simulink model "DTMF_Telefonie_Project_Crehul_Hornai"  (R2018b)
settings: Solver=VariableStepAuto  StartTime=0.0  StopTime=100  RelTol=1e-3
undefined symbols (not defined in the file): fdesignblkfcn, gcbh
libraries: simulink x12, dspfdesign x7
(part 2 of 4)

== system DTMF_Telefonie_Project_Crehul_Hornai/DTMF Detector and Decoder/Subsystem/1477Hz Bandpass Filter ==
  In : Inport
  Generated Filter Block : DiscreteFir  Tag=BlockMethodSubSystem  Coefficients=[0.000678764862504704263 0.000804373453114689695 -0.000424094188809401567 0.000167209003489621763 -0.000242270760367763161 4.6470921147658429e-05 6.95206164852695159e-06 0.000136313750795735581 5.73971292841914723e-05 -1.08891135695370588e-05 -0.00010807231843965948 -0.000100678178529028895 -2.39139709179673077e-05 8.22719619307408709e-05 0.000121322031372226961 6.67195498408230687e-05 -4.54322205964575315e-05 -0.000123546441105899405 -0.000105769303813425504 -1.47191102267772017e-06 0.000106642780553394814 0.000132557583534852327 5.13511648645235529e-05 -7.37028057411876717e-05 -0.000143736658268125549 -9.92899356923174822e-05 2.59446525748383179e-05 0.000134079459699696767 0.000136741672296518922 3.01685686462495675e-05 -0.000104187130503145776 -0.000158239484929200433 -8.67404980072451152e-05 5.74174071110912943e-05 0.000158308721508832297 0.000134444966268375916 1.8284919510189266e-06 -0.000134817878355808192 -0.000167440391573942578 -6.55512682525988006e-05 9.14538284917498345e-05 0.000178631042614973241 0.000123874664584542075 -3.05242741126250487e-05 -0.000164714196852270645 -0.000169025187109667335 -3.7701329655403246e-05 0.000126528809334661456 0.000192066158003905601 0.000105799063218011509 -6.79533803345053634e-05 -0.000189773665441093139 -0.000161994152014295189 -3.95880851204494406e-06 0.000160060971546786227 0.000199138171986074433 7.8476057786001311e-05 -0.000105980075455429975 -0.000209346483238170194 -0.000146288941368850336 3.45550752056478314e-05 0.000190352324485544306 0.000196109461443976646 4.54400805598609726e-05 -0.000144484544870355494 -0.000220406187691344485 -0.000121964269468380565 7.58152294997171006e-05 0.00021488709301901044 0.000184083746180164782 5.93982545919963592e-06 -0.000178893689660710982 -0.000223002253409260078 -8.89183572636694994e-05 0.000116458060922216113 0.000231657134855096621 0.000162204277360463367 -3.64712308000864505e-05 -0.000208119503375310717 -0.000214664067654908195 -5.02598167574192737e-05 0.000155096389684706779 0.000238098225791522154 0.000132194115690055384 -7.99892046078015499e-05 -0.000228623801064775992 -0.000196701983237502565 -7.34495975451181574e-06 0.000187575168349489452 0.000234483903146764146 9.4383718966663515e-05 -0.000120350652338928072 -0.00023975742986282909 -0.000168765668975382659 3.62796888475293202e-05 0.000212334960261702623 0.000219332269412665605 5.26832536310174303e-05 -0.000155766501238902705 -0.000239303864982351108 -0.000133517294274330045 7.82814639436078472e-05 0.000226012067649557441 0.000194762278839820174 8.6425324803695875e-06 -0.000182112956171246246 -0.000227689150524581184 -9.25658528431953353e-05 0.000114226987622273067 0.000228657881637320173 0.000161021804288971051 -3.27910592299296682e-05 -0.000198224146624526205 -0.000204801318833720825 -4.99979298250496137e-05 0.000141908848976985986 0.000218455210176687897 0.000122065229315672548 -6.91953924481208526e-05 -0.000201291882550297093 -0.00017324112862875953 -8.77095916717294567e-06 0.000157781157199081944 0.000197131314976748805 8.00474503860715107e-05 -9.56231695524905126e-05 -0.000192124851322154596 -0.000134438958140752031 2.573733020283216e-05 0.000161008172845363701 0.000165063910650344644 4.07422142637717342e-05 -0.000110735349115864516 -0.000169367326537080923 -9.38498835634843289e-05 5.12370725678648956e-05 0.000149182379205609061 0.000126667649759154262 7.12439653057449739e-06 -0.00011079587869896961 -0.000136065294631048609 -5.48549739532533474e-05 6.29644289637935114e-05 0.000123760079219049609 8.49249951684299779e-05 -1.54504623116251492e-05 -9.51766421847845007e-05 -9.47953617583736398e-05 -2.27547304877335002e-05 5.8641671409375264e-05 8.59013188943345395e-05 4.53598683612078338e-05 -2.32918846142151498e-05 -6.37716681334422452e-05 -5.01656451408910315e-05 -2.43092022642965935e-06 3.63407014523718219e-05 3.92725335328120324e-05 1.30810954317975205e-05 -1.28066060299382271e-05 -1.84926479954187692e-05 -7.304766428425577e-06 1.06809246101379103e-06 ...(+19715 chars)]  InputProcessing=Columns as channels (frame based)
  Out : Outport
  wires:
  In/1 -> Generated Filter Block/1
  Generated Filter Block/1 -> Out/1

== system DTMF_Telefonie_Project_Crehul_Hornai/DTMF Detector and Decoder/Subsystem1/697Hz Bandpass Filter ==
  In : Inport
  Generated Filter Block : DiscreteFir  Tag=BlockMethodSubSystem  Coefficients=[-0.000394264594047649903 0.000774744811871758469 0.000427421881547907574 0.000281317478265080809 0.000190859822015726602 0.000103220041783864784 6.02395013947904024e-06 -9.38100617318130052e-05 -0.000181273083465624681 -0.000239401956619517684 -0.000254792159022771292 -0.000220736657481967845 -0.000140010751800439078 -2.4597335521758199e-05 0.000105253535811033959 0.000225097179614547549 0.000310164874170040642 0.000340985600688686213 0.000307015089505039123 0.000210115053645176168 6.44184314711238363e-05 -0.000104781527711556485 -0.000266062164349415277 -0.000386865749964367643 -0.000440675160994910455 -0.000411889611254364263 -0.000300580253768110203 -0.000122627077751380682 9.1344109890286864e-05 0.000302046872857163976 0.00046766859725355718 0.00055304385098083747 0.000535877947879521109 0.000413278082280569344 0.00020215757186176192 -6.13660267820909441e-05 -0.000329454718671672107 -0.000549541536983108874 -0.000676281823529430452 -0.000678751503028325273 -0.000549882077295554632 -0.000306193937980755364 1.02868595120332844e-05 0.000343691861983609626 0.00062808600222025255 0.000807734386134440125 0.000840107722215793448 0.000711077835160514376 0.00043916359257390906 6.56484195848901941e-05 -0.000339386541605346569 -0.000699565032775093919 -0.000943446141897278452 -0.00101820431616139609 -0.000899182966261597317 -0.000600200646850151736 -0.000170517840281379085 0.000312538832414332025 0.000758822687122101872 0.0010802524341631595 0.00120898266532983999 0.00111051976159609904 0.000793394831748578649 0.000308499665591947174 -0.000257936638108287298 -0.000800440291611864891 -0.00121303423350785995 -0.00141055855900055994 -0.00134524092784002913 -0.00101838262461309689 -0.000481505832679848702 0.000170790574874636971 0.000817909483250049696 0.00133483161593174623 0.00161676542535599157 0.00159961742467604998 0.00127461301979677551 0.000691711243999674108 -4.71855876618361886e-05 -0.00080631435833903762 -0.00144039387824669964 -0.00182281431995734585 -0.00187029926250970903 -0.00156100928321011522 -0.000940771614561606434 -0.00011710236537692959 0.000759512530315526032 0.00152262968074125173 0.00202194341881048673 0.00215171567088028818 0.00187453924518769864 0.00122820467004980567 0.000324811393669725769 -0.000672404770145742462 -0.00157505271903591692 -0.00220690302712525047 -0.00243817778597354897 -0.00221097458378263128 -0.00155335621023871152 -0.000577564193468575716 0.000540169773833136524 0.00159066822638551726 0.002370740997611451 0.00272233680065818873 0.0025650876086355549 0.00191329848025059354 0.000876377433019636548 -0.000359376878288369072 -0.00156355101099926773 -0.00250508324075643211 -0.00299630406661315334 -0.00293046990732039785 -0.00230391680503208313 -0.00122021264083055315 0.000126882061588719919 0.00148750434151111144 0.00260238815577148877 0.00325186557664835412 0.00329946697874916638 0.00271977574669979467 0.00160667721650968229 0.000158206661703232473 -0.00135814406868356333 -0.00265520189891188009 -0.00347996795138794893 -0.00366335837877724288 -0.00315415662057392165 -0.00203222836275578208 -0.000496059675174653574 0.00117170261385296732 0.00265686177459320376 0.0036720160005349555 0.00401306165529105845 0.00359898263542247519 0.00249140500652611898 0.000884955608487839203 -0.00092590165413497657 -0.0026012069990905707 -0.0038194990314259613 -0.00433869741609792768 -0.00404519073742530804 -0.00297723106091718958 -0.00132126938878718249 0.000620064148982378549 0.00248383801806922096 0.00391434016938745598 0.0046308674195702634 0.00448293486091789518 0.00348162421875347888 0.00180024560270603527 -0.000255105110608400847 -0.00230126355280119241 -0.00394951765388701446 -0.00487964953703672391 -0.00490178117438651913 -0.00399508998313839649 -0.00231481267956316298 -0.000166078513184513823 0.00205175855072361893 0.00391922279101129811 0.00507614101092128574 0.0052909328979446283 0.00450715066155292585 0.00285690180509721092 0.00063894139925937119 -0.00173553441141433592 -0.00381895652133022994 ...(+7766 chars)]  InputProcessing=Columns as channels (frame based)
  Out : Outport
  wires:
  In/1 -> Generated Filter Block/1
  Generated Filter Block/1 -> Out/1
